simulink model "Simulink_Beta_oscillations_model"  (R2025a)
settings: Solver=FixedStepAuto  StartTime=0.0  StopTime=10  FixedStep=1e-5  MaxStep=0.01  RelTol=1e-5
settings Model: Creator=enash  LastModifiedBy=Student
settings OptimizationCC: ReuseModelBlockBuffer=off
settings RTWCC: GPUComputeCapability=3.5

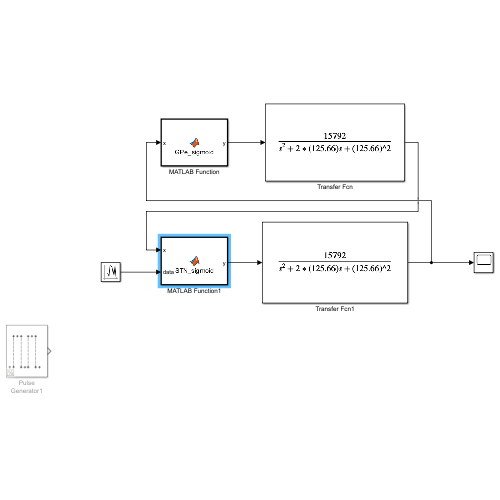
[thumbnail: Simulink's stored preview of the top-level diagram]
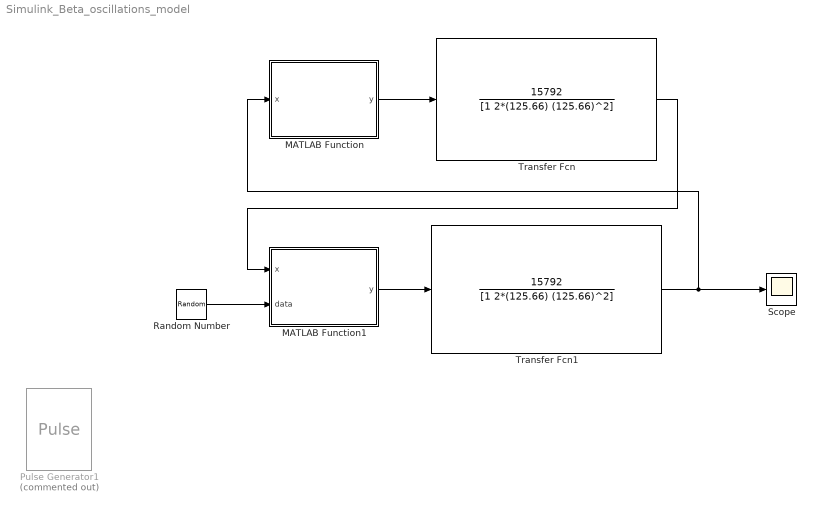
== system Simulink_Beta_oscillations_model ==
  MATLAB Function : MATLAB Function  TreatAsAtomicUnit=on
  MATLAB Function1 : MATLAB Function  TreatAsAtomicUnit=on
  Pulse Generator1 : DiscretePulseGenerator  Commented=on  Amplitude=0.1  Period=2e6  PulseWidth=2e2  SampleTime=1e-5
  Random Number : RandomNumber  Variance=1e-6  SampleTime=1e-5
  Scope : Scope
      settings: ActiveDisplayYMinimum=-0.15125538506255762  ActiveDisplayYMaximum=0.15125537083968055
  Transfer Fcn : TransferFcn  Numerator=[15792]  Denominator=[1 2*(125.66) (125.66)^2]
  Transfer Fcn1 : TransferFcn  Numerator=[15792]  Denominator=[1 2*(125.66) (125.66)^2]
  wires:
  MATLAB Function/1(y) -> Transfer Fcn/1
  MATLAB Function1/1(y) -> Transfer Fcn1/1
  Transfer Fcn1/1 -> Scope/1, MATLAB Function/1(x)
  Transfer Fcn/1 -> MATLAB Function1/1(x)
  Random Number/1 -> MATLAB Function1/2(data)

== matlab function Simulink_Beta_oscillations_model/MATLAB Function1 ==
  data: x input; y output; data input
function y = STN_sigmoid(x, data)

g = 1.5; % Sharpness parameter for GPe
y = (2/pi)*atan((data-x)/g);

end

== matlab function Simulink_Beta_oscillations_model/MATLAB Function ==
  data: x input; y output
% function y = GPe_sigmoid(x)
% function y = GPe_sigmoid(x)
% function y = GPe_sigmoid(x)
%     % Create h values from 1 to 0.01 and back to 1
%     h_values = [1:-0.25:0.01, 0.01:0.25:1]; 
%     num_h = length(h_values); % Number of h values
% 
%     % Preallocate output y as a 1D array with size based on h_values
%     y = zeros(num_h, 1); % One output value for each h
% 
%     % Loop through each value of h
%     for i = 1:num_h
%         h = h_values(i);
%         % Compute the average of the sigmoid function for the current h
%         y(i) = mean((2/pi) * atan(x/h)); % Compute mean for current h
%     end
% end


function y = GPe_sigmoid(x)

% h is the sharpness parameter of the GPe sigmoid function
% if t >= 0.25 && t <= 1.0
%     h = 1.0;
% elseif t >= 2.0 && t <= 2.5
%     h = 1.0;
% elseif t >= 4 && t <= 6
%     h = 1.0;
% else 
%     h = 0.1;
% end

h = 0.01;

% Calculate the output using the sigmoid function
y = (2/pi)*atan(x/h); 
end
